simulink model "vehicle_model2"  (R2017b)
settings: Solver=VariableStepAuto  StartTime=0.0  StopTime=100  RelTol=1e-3
values from neighbouring files (symbols this model uses):
  d = 0.10    (= 0.1)    [main.m]
  R = 0.056/2    (= 0.028)    [main.m]
undefined symbols (not defined in the file or in its folder): lkk, lP12, lP1P2, q1, q2, rkk, rP12, rP1P2
libraries: simulink x3, dspstat3 x2
settings Model: Creator=hoh  LastModifiedBy=Ale

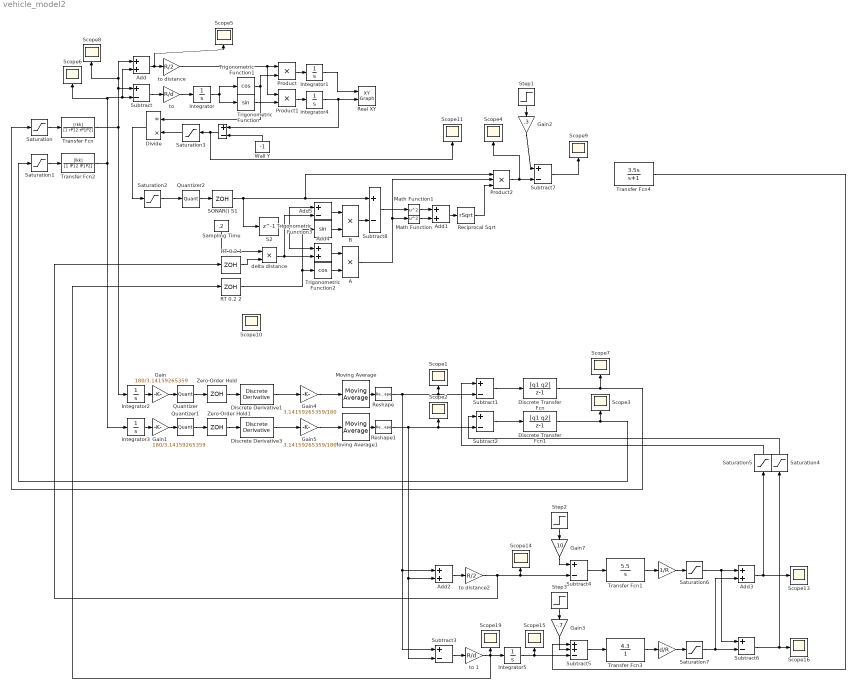
== system vehicle_model2 ==
  " " : Gain  Gain=1/R
  "   " : Sum  Inputs=+-
  "       " : Gain  Gain=d/R
  A : Product
  Add{,1..4} (5 alike) : Sum
  Add5 : Sum  Inputs=+-
  B : Product
  Discrete Transfer Fcn : DiscreteTransferFcn  Numerator=[q1 q2]  Denominator=[1 -1]
  Discrete Transfer Fcn1 : DiscreteTransferFcn  Numerator=[q1 q2]  Denominator=[1 -1]
  Discrete Derivative1 : simulink/Discrete/Discrete Derivative  gainval=1  ICPrevScaledInput=0  OutMin=[]  OutMax=[]  OutDataType=fixdt(1, 16)  OutScaling=2^-10  DoSatur=off
  Discrete Derivative3 : simulink/Discrete/Discrete Derivative  gainval=1  ICPrevScaledInput=0  OutMin=[]  OutMax=[]  OutDataType=fixdt(1, 16)  OutScaling=2^-10  DoSatur=off
  Divide : Product  Inputs=/*
  Gain : Gain  Gain=180/3.14159265359
  Gain1 : Gain  Gain=180/3.14159265359
  Gain2 : Gain  Gain=.3
  Gain3 : Gain  Gain=-.7
  Gain4 : Gain  Gain=3.14159265359/180
  Gain5 : Gain  Gain=3.14159265359/180
  Gain7 : Gain  Gain=.10
  Integrator{,1..5} (6 alike) : Integrator
  Math Function : Math  Operator=square  SaturateOnIntegerOverflow=on
  Math Function1 : Math  Operator=square  SaturateOnIntegerOverflow=on
  Moving Average : dspstat3/Moving Average  Method=Exponential weighting  SpecifyWindowLength=on  WindowLength=3  ForgettingFactor=.7  SimulateUsing=Code generation
  Moving Average1 : dspstat3/Moving Average  Method=Exponential weighting  SpecifyWindowLength=on  WindowLength=4  ForgettingFactor=0.7  SimulateUsing=Code generation
  Product : Product
  Product1 : Product
  Product2 : Product  Inputs=3
  Quantizer : Quantizer  QuantizationInterval=1
  Quantizer1 : Quantizer  QuantizationInterval=1
  Quantizer2 : Quantizer  QuantizationInterval=.01
  RT 0.2 1 : ZeroOrderHold  SampleTime=0.2
  RT 0.2 2 : ZeroOrderHold  SampleTime=0.2
  Real XY : simulink/Sinks/XY Graph  xmin=0  xmax=5  ymin=-5  ymax=1  st=-1
  Reciprocal Sqrt : Sqrt  Operator=rSqrt  SaturateOnIntegerOverflow=on
  Reshape : Reshape
  Reshape1 : Reshape
  "S2 " : Delay  DelayLength=1  InitialCondition=0
  "SONAR() S1 " : ZeroOrderHold  SampleTime=0.2
  Sampling Time : Constant  Value=.2
  Saturation : Saturate  UpperLimit=100  LowerLimit=0
  Saturation1 : Saturate  UpperLimit=100  LowerLimit=0
  Saturation2 : Saturate  UpperLimit=1.5  LowerLimit=.02
  Saturation3 : Saturate  UpperLimit=100  LowerLimit=0
  Saturation4 : Saturate  UpperLimit=12  LowerLimit=0
  Saturation5 : Saturate  UpperLimit=12  LowerLimit=0
  Saturation6 : Saturate  UpperLimit=12  LowerLimit=0
  Saturation7 : Saturate  UpperLimit=12  LowerLimit=-12
  Scope{1..11,13..16,19} (16 alike) : Scope
  Step1 : Step  Time=0  SampleTime=0
  Step2 : Step  Time=0  SampleTime=0
  Step3 : Step  Time=3  SampleTime=0
  Subtract{,1..4,6..8} (8 alike) : Sum  Inputs=+-
  Subtract5 : Sum  Inputs=++-
  Transfer Fcn : TransferFcn  Numerator=[rkk]  Denominator=[1 rP12 rP1P2]
  Transfer Fcn1 : TransferFcn  Numerator=[5.5]  Denominator=[1 0]
  Transfer Fcn2 : TransferFcn  Numerator=[lkk]  Denominator=[1 lP12 lP1P2]
  Transfer Fcn3 : TransferFcn  Numerator=[4.3]  Denominator=[1]
  Transfer Fcn4 : TransferFcn  Numerator=[3.5 0]  Denominator=[1 1]
  Trigonometric Function : Trigonometry
  Trigonometric Function1 : Trigonometry  Operator=cos
  Trigonometric Function2 : Trigonometry  Operator=cos
  Trigonometric Function3 : Trigonometry
  Wall Y : Constant  Value=-1
  Zero-Order Hold : ZeroOrderHold  SampleTime=0.005
  Zero-Order Hold1 : ZeroOrderHold  SampleTime=0.005
  delta distance : Product
  "to " : Gain  Gain=R/d
  to 1 : Gain  Gain=R/d
  to distance : Gain  Gain=R/2
  to distance2 : Gain  Gain=R/2
  wires:
  Subtract/1 -> "to "/1
  Integrator/1 -> Trigonometric Function/1, Trigonometric Function1/1
  to distance/1 -> Product1/1, Product/1
  Product/1 -> Integrator1/1
  Integrator1/1 -> Real XY/1
  Product1/1 -> Integrator4/1
  Add/1 -> Scope5/1, to distance/1
  "to "/1 -> Integrator/1
  Integrator2/1 -> Gain/1
  Quantizer/1 -> Zero-Order Hold/1
  Quantizer1/1 -> Zero-Order Hold1/1
  Gain1/1 -> Quantizer1/1
  Integrator3/1 -> Gain1/1
  Trigonometric Function/1 -> Product1/2
  Saturation1/1 -> Transfer Fcn2/1
  Saturation/1 -> Transfer Fcn/1
  Quantizer2/1 -> "SONAR() S1 "/1
  Divide/1 -> Saturation2/1
  Saturation2/1 -> Quantizer2/1
  Integrator4/1 -> "   "/1, Real XY/2
  Trigonometric Function1/1 -> Product/2, Divide/1
  Transfer Fcn2/1 -> Integrator3/1, Scope6/1, Subtract/2, Add/2
  Zero-Order Hold/1 -> Discrete Derivative1/1
  Zero-Order Hold1/1 -> Discrete Derivative3/1
  Wall Y/1 -> "   "/2
  "   "/1 -> Scope11/1, Saturation3/1
  Saturation3/1 -> Divide/2
  Add3/1 -> Scope13/1, Saturation5/1
  Discrete Derivative1/1 -> Gain4/1
  Moving Average/1 -> Reshape/1
  Discrete Derivative3/1 -> Gain5/1
  Moving Average1/1 -> Reshape1/1
  Gain4/1 -> Moving Average/1
  Gain5/1 -> Moving Average1/1
  Gain/1 -> Quantizer/1
  Subtract1/1 -> Discrete Transfer Fcn/1
  Subtract2/1 -> Discrete Transfer Fcn1/1
  Discrete Transfer Fcn/1 -> Saturation/1, Scope7/1
  Discrete Transfer Fcn1/1 -> Saturation1/1, Scope3/1
  Reshape/1 -> Add2/1, Subtract3/1, Subtract1/2, Scope1/1
  Reshape1/1 -> Add2/2, Subtract3/2, Subtract2/2, Scope2/1
  Transfer Fcn/1 -> Scope8/1, Add/1, Subtract/1, Integrator2/1
  Subtract6/1 -> Scope16/1, Saturation4/1
  Add2/1 -> to distance2/1
  Subtract3/1 -> to 1/1
  Step3/1 -> Gain3/1
  Step2/1 -> Gain7/1
  Subtract4/1 -> Transfer Fcn1/1
  to 1/1 -> RT 0.2 2/1, Scope19/1, Integrator5/1
  to distance2/1 -> RT 0.2 1/1, Subtract4/2, Scope14/1
  Gain7/1 -> Subtract4/1
  Gain3/1 -> Subtract5/2
  Transfer Fcn1/1 -> " "/1
  Subtract5/1 -> Transfer Fcn3/1
  "       "/1 -> Saturation7/1
  " "/1 -> Saturation6/1
  Saturation4/1 -> Subtract2/1
  Saturation5/1 -> Subtract1/1
  Integrator5/1 -> Subtract5/3, Scope15/1
  Saturation6/1 -> Add3/1, Subtract6/1
  Saturation7/1 -> Add3/2, Subtract6/2
  Transfer Fcn3/1 -> "       "/1
  Step1/1 -> Gain2/1
  Gain2/1 -> Subtract7/1
  Subtract7/1 -> Scope9/1
  Transfer Fcn4/1 -> Subtract5/1
  Product2/1 -> Scope4/1, Subtract7/2
  "SONAR() S1 "/1 -> "S2 "/1, Subtract8/1, Product2/1
  Trigonometric Function2/1 -> A/2
  Add4/1 -> A/1
  Sampling Time/1 -> delta distance/1
  "S2 "/1 -> Add5/1, Add4/1
  A/1 -> Product2/2, Math Function/1
  Reciprocal Sqrt/1 -> Product2/3
  Add1/1 -> Reciprocal Sqrt/1
  Subtract8/1 -> Math Function1/1
  Add5/1 -> B/1
  Trigonometric Function3/1 -> B/2
  B/1 -> Subtract8/2
  Math Function/1 -> Add1/2
  Math Function1/1 -> Add1/1
  RT 0.2 2/1 -> Trigonometric Function3/1, Trigonometric Function2/1
  RT 0.2 1/1 -> delta distance/2
  delta distance/1 -> Add4/2, Add5/2
